simulink model "work"  (Simulink 7.5)
settings: Solver=ode45  StartTime=0.0  StopTime=30.0  RelTol=1e-3
libraries: cstblocks x1
settings Model: Creator=davito  LastModifiedBy=davito

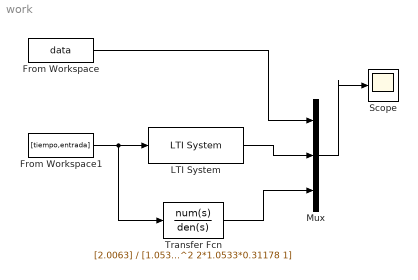
== system work ==
  From Workspace : FromWorkspace  VariableName=data  SampleTime=0.00390600000000000
  From Workspace1 : FromWorkspace  VariableName=[tiempo,entrada]  SampleTime=0.00390600000000000
  LTI System : cstblocks/LTI System  SystemSampleTime=-1  sys=tf(2.0063,[1.053^2 2*0.31178*1.053 1])  IC=[]
  Mux : Mux  Inputs=3
  Scope : Scope
  Transfer Fcn : TransferFcn  Numerator=[2.0063]  Denominator=[1.0533^2 2*1.0533*0.31178 1]
  wires:
  From Workspace/1 -> Mux/1
  LTI System/1 -> Mux/2
  Mux/1 -> Scope/1
  From Workspace1/1 -> LTI System/1, Transfer Fcn/1
  Transfer Fcn/1 -> Mux/3
